simulink model "IdealScheme_soft_start"  (R2021b)
settings: Solver=VariableStepAuto  StartTime=0.0  StopTime=10  RelTol=1e-3
libraries: spsDiodeLib x7, spsMeanLib x5, spsSeriesRLCBranchLib x4, spsCurrentMeasurementLib x2, spsVoltageMeasurementLib x2, spsDCMachineLib x1, spsDCVoltageSourceLib x1, spsGroundLib x1, spsIGBTLib x1, slpidlib x1, spsThreePhaseSourceLib x1, spspowerguiLib x1
settings Model: Creator=kkaya674  LastModifiedBy=kkaya674
settings SolverCC: ZeroCrossAlgorithm=Adaptive
settings DebuggingCC: IgnoredZcDiagnostic=none

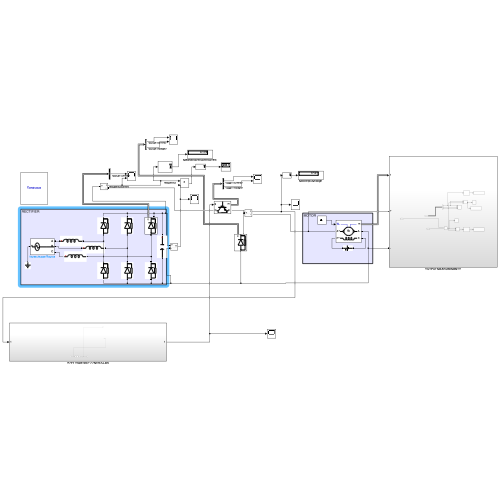
[thumbnail: Simulink's stored preview of the top-level diagram]
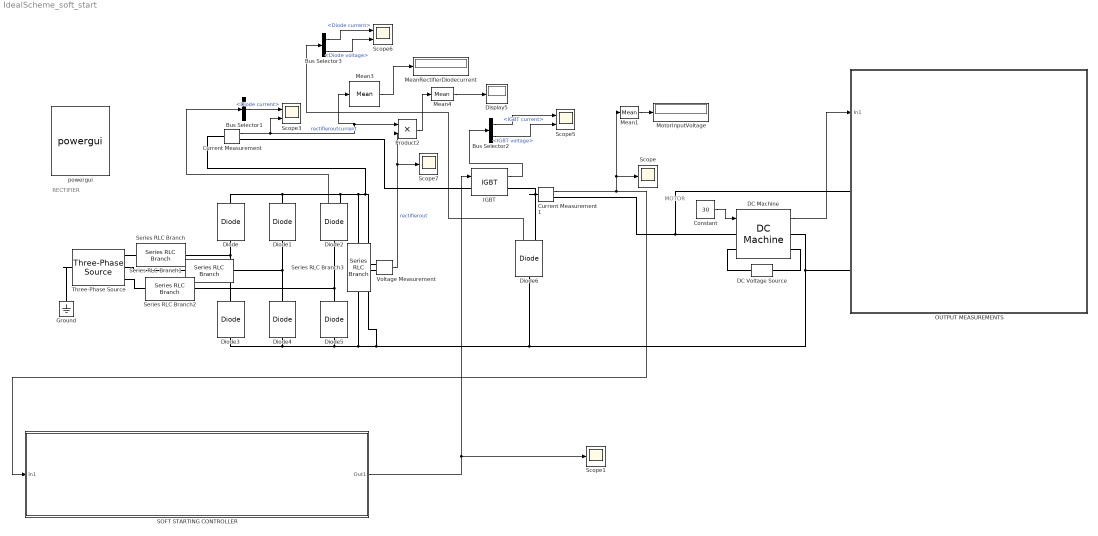
== system IdealScheme_soft_start ==
  note: MOTOR
  note: RECTIFIER
  Bus Selector1 : BusSelector  OutputSignals=Diode current
  Bus Selector2 : BusSelector  OutputSignals=IGBT current,IGBT voltage
  Bus Selector3 : BusSelector  OutputSignals=Diode current,Diode voltage
  Constant : Constant  Value=30
  Current Measurement : spsCurrentMeasurementLib/Current Measurement  PhasorSimulation=off  OutputType=Complex  PSBequivalent=0
  Current Measurement1 : spsCurrentMeasurementLib/Current Measurement  PhasorSimulation=off  OutputType=Complex  PSBequivalent=0
  DC Machine : spsDCMachineLib/DC Machine  PresetModel=No  MechanicalLoad=Torque TL  FieldType=Wound  ShowDetailedParameters=on  MeasurementBus=off  RLa=[0.8 12.5e-3]  RLf=[210 23]  Laf=1.8  MachineConstant=Torque constant (N.m/A)  Ke=1.8  Kt=1.8  J=1  Bm=0  Tf=0  w0=0  Ifinit=1.04761904756944  TsPowergui=0  TsBlock=-1
  DC Voltage Source : spsDCVoltageSourceLib/DC Voltage Source  Amplitude=220  Measurements=None
  Diode{,1,3..5} (5 alike) : spsDiodeLib/Diode  Ron=0.001  Lon=0  Vf=0.8  IC=0  UseSnubber=0  Rs=500  Cs=250e-9  Measurements=off
  Diode2 : spsDiodeLib/Diode  Ron=0.001  Lon=0  Vf=0.8  IC=0  UseSnubber=0  Rs=500  Cs=250e-9  Measurements=on
  Diode6 : spsDiodeLib/Diode  Ron=0.001  Lon=0  Vf=0.8  IC=0  UseSnubber=0  Rs=500  Cs=250e-9  Measurements=on
  Display5 : Display
  Ground : spsGroundLib/Ground  LConnTagsString=a
  IGBT : spsIGBTLib/IGBT  Ron=0.001  Lon=0  Vf=1  Tf=1e-6  Tt=2e-6  IC=0  Rs=1e5  Cs=inf  Measurements=on
  Mean1 : spsMeanLib/Mean  Freq=60  Vinit=0  Ts=0
  Mean3 : spsMeanLib/Mean  Freq=50  Vinit=0  Ts=0
  Mean4 : spsMeanLib/Mean  Freq=50  Vinit=0  Ts=0
  MeanRectifierDiodecurrent : Display
  MotorInputVoltage : Display
  OUTPUT MEASUREMENTS : Subsystem
  Product2 : Product
  SOFT STARTING CONTROLLER : Subsystem
  Scope : Scope
  Scope1 : Scope
  Scope3 : Scope  NumInputPorts=2
  Scope5 : Scope  NumInputPorts=2
  Scope6 : Scope  NumInputPorts=2
  Scope7 : Scope
  Series RLC Branch : spsSeriesRLCBranchLib/Series RLC Branch  LConnTagsString=__new0  RConnTagsString=__new0  BranchType=L  Resistance=1  Inductance=0.05e-3  SetiL0=off  InitialCurrent=0  Capacitance=1e-6  Setx0=off  InitialVoltage=0  Measurements=None
  Series RLC Branch1 : spsSeriesRLCBranchLib/Series RLC Branch  LConnTagsString=__new0  RConnTagsString=__new0  BranchType=L  Resistance=1  Inductance=0.05e-3  SetiL0=off  InitialCurrent=0  Capacitance=1e-6  Setx0=off  InitialVoltage=0  Measurements=None
  Series RLC Branch2 : spsSeriesRLCBranchLib/Series RLC Branch  LConnTagsString=__new0  RConnTagsString=__new0  BranchType=L  Resistance=1  Inductance=0.05e-3  SetiL0=off  InitialCurrent=0  Capacitance=1e-6  Setx0=off  InitialVoltage=0  Measurements=None
  Series RLC Branch3 : spsSeriesRLCBranchLib/Series RLC Branch  LConnTagsString=__new0  RConnTagsString=__new0  BranchType=C  Resistance=1  Inductance=1e-3  SetiL0=off  InitialCurrent=0  Capacitance=470e-6  Setx0=off  InitialVoltage=0  Measurements=None
  Three-Phase Source : spsThreePhaseSourceLib/Three-Phase Source  InternalConnection=Yn  VoltagePhases=off  Voltage=166  PhaseAngle=0  Voltage_phases=[25e3 25e3 25e3]/sqrt(3)  PhaseAngles_phases=[0 -120 +120]  Frequency=50  NonIdealSource=off  SpecifyImpedance=off  Resistance=0.8929  Inductance=16.58e-3  ShortCircuitLevel=100e6  BaseVoltage=25e3  XRratio=7  BusType=swing  Pref=10e3  Qref=0  Prefabc=[10e3, 10e3, 10e3]  Qrefabc=[0, 0, 0]  Qmin=-inf  Qmax=inf
  Voltage Measurement : spsVoltageMeasurementLib/Voltage Measurement  PhasorSimulation=off  OutputType=Complex  PSBequivalent=0
  powergui : spspowerguiLib/powergui  Priority=1  SimulationMode=Continuous  SampleTime=50e-6  frequency=60  Iterations=50  frequencyindice=0  Pbase=100e6  ErrMax=1e-4  UnitsV=kV  UnitsW=MW  buscounter=0  FunctionMessages=off  echomessages=off  EnableUseOfTLC=off  CurrentSourceSwitches=off  DisableSnubberDevices=off  DisableRonSwitches=off  DisableVfSwitches=off  DisplayEquations=off  AutomaticDiscreteSolvers=off  SolverType=Tustin/Backward Euler (TBE)  Interpol=off  ExternalGateDelay=off  methode=off  Ts=100  x0status=blocks  SPID=on  SwTol=0  HookPort=off  NonlinearTolerance=1e-4  nMaxIteration=100  ContinueOnMaxIteration=off  RestoreLinks=warning  ResistiveCurrentMeasurement=off  Frange=[0:2:500]  Ylog=off  Xlog=on  ShowGrid=off  save=off  variable=ZData  structure=0  ZoomFFT=off  StartTime=0.0  cycles=1  DisplayStyle=1  fundamental=60  FreqAxis=off  MaxFrequency=1000  frequencyindicesteady=1  RmsSteady=1  display=off
  wires:
  Voltage Measurement/1 -> Scope7/1, Product2/2  "rectifierout"
  Mean1/1 -> MotorInputVoltage/1
  IGBT/1 -> Bus Selector2/1
  Bus Selector2/1 -> Scope5/1  "<IGBT current>"
  Bus Selector2/2 -> Scope5/2  "<IGBT voltage>"
  Diode6/1 -> Bus Selector3/1
  Bus Selector3/1 -> Scope6/1  "<Diode current>"
  Bus Selector3/2 -> Scope6/2  "<Diode voltage>"
  Constant/1 -> DC Machine/1
  Diode2/1 -> Bus Selector1/1
  Bus Selector1/1 -> Scope3/1  "<Diode current>"
  Current Measurement/1 -> Scope3/2, Mean3/1, Product2/1  "rectifieroutcurrent"
  Mean3/1 -> MeanRectifierDiodecurrent/1
  Product2/1 -> Mean4/1
  Mean4/1 -> Display5/1
  Current Measurement1/1 -> Mean1/1, Scope/1, SOFT STARTING CONTROLLER/1(In1)
  DC Machine/1 -> OUTPUT MEASUREMENTS/1(In1)
  SOFT STARTING CONTROLLER/1(Out1) -> Scope1/1, IGBT/1
  connections:
  Diode3/RConn1 -- Series RLC Branch/RConn1 -- Diode/LConn1
  Diode4/RConn1 -- Series RLC Branch1/RConn1 -- Diode1/LConn1
  Diode5/RConn1 -- Series RLC Branch2/RConn1 -- Diode2/LConn1
  Current Measurement1/RConn1 -- OUTPUT MEASUREMENTS/LConn1 -- DC Machine/LConn1
  Diode/RConn1 -- Series RLC Branch3/LConn1 -- Voltage Measurement/LConn1 -- Current Measurement/LConn1 -- Diode2/RConn1 -- Diode1/RConn1
  Three-Phase Source/LConn1 -- Ground/LConn1
  DC Voltage Source/RConn1 -- DC Machine/LConn2
  DC Voltage Source/LConn1 -- DC Machine/RConn2
  IGBT/RConn1 -- Current Measurement1/LConn1 -- Diode6/RConn1
  IGBT/LConn1 -- Current Measurement/RConn1
  Three-Phase Source/RConn1 -- Series RLC Branch/LConn1
  Three-Phase Source/RConn2 -- Series RLC Branch1/LConn1
  Three-Phase Source/RConn3 -- Series RLC Branch2/LConn1
  Diode6/LConn1 -- OUTPUT MEASUREMENTS/LConn2 -- DC Machine/RConn1 -- Voltage Measurement/LConn2 -- Series RLC Branch3/RConn1 -- Diode4/LConn1 -- Diode3/LConn1 -- Diode5/LConn1

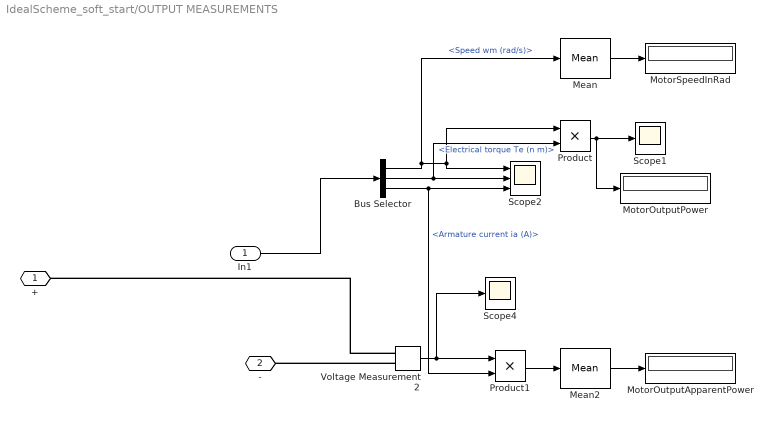
== system IdealScheme_soft_start/OUTPUT MEASUREMENTS ==
  In1 : Inport
  Bus Selector : BusSelector  OutputSignals=Speed wm (rad/s),Electrical torque Te (n m),Armature current ia (A)
  Mean : spsMeanLib/Mean  Freq=60  Vinit=0  Ts=0
  Mean2 : spsMeanLib/Mean  Freq=50  Vinit=0  Ts=0
  MotorOutputApparentPower : Display
  MotorOutputPower : Display
  MotorSpeedInRad : Display
  Product : Product
  Product1 : Product
  Scope1 : Scope
  Scope2 : Scope  NumInputPorts=3
  Scope4 : Scope
  Voltage Measurement2 : spsVoltageMeasurementLib/Voltage Measurement  PhasorSimulation=off  OutputType=Complex  PSBequivalent=0
  + : PMIOPort  Side=Left
  - : PMIOPort  Port=2  Side=Left
  wires:
  Voltage Measurement2/1 -> Product1/1, Scope4/1
  Bus Selector/2 -> Product/2, Scope2/2  "<Electrical torque Te (n m)>"
  In1/1 -> Bus Selector/1
  Mean/1 -> MotorSpeedInRad/1
  Product/1 -> MotorOutputPower/1, Scope1/1
  Product1/1 -> Mean2/1
  Bus Selector/1 -> Mean/1, Scope2/1, Product/1  "<Speed wm (rad/s)>"
  Mean2/1 -> MotorOutputApparentPower/1
  Bus Selector/3 -> Product1/2, Scope2/3  "<Armature current ia (A)>"
  connections:
  Voltage Measurement2/LConn2 -- -/RConn1
  Voltage Measurement2/LConn1 -- +/RConn1

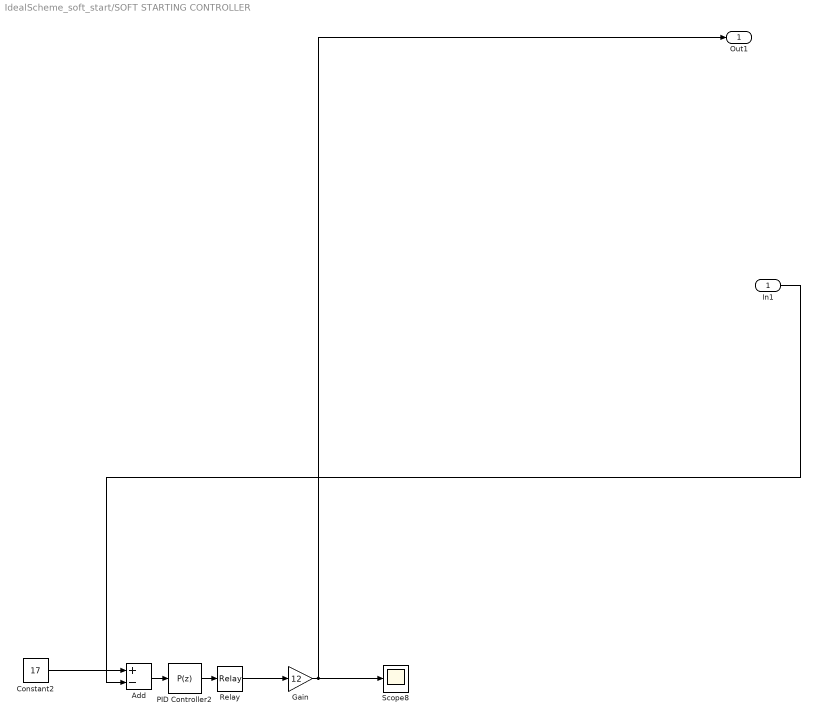
== system IdealScheme_soft_start/SOFT STARTING CONTROLLER ==
  In1 : Inport
  Add : Sum  Inputs=+-
  Constant2 : Constant  Value=17
  Gain : Gain  Gain=12
  PID Controller2 : slpidlib/PID Controller  Controller=P  Form=Parallel  TimeDomain=Discrete-time  UseExternalTs=off  SampleTime=-1  IntegratorMethod=Forward Euler  FilterMethod=Forward Euler  ControllerParametersSource=internal  P=1  I=0  D=0  UseFilter=on  N=100  TunerSelectOption=Transfer Function Based (PID Tuner App)  InitialConditionSource=internal  InitialConditionForIntegrator=0  InitialConditionForFilter=0  DifferentiatorICPrevScaledInput=0  ExternalReset=none  TrackingMode=off  Kt=1  LimitOutput=off  SatLimitsSource=internal  UpperSaturationLimit=inf  LowerSaturationLimit=-inf  LinearizeAsGain=on  AntiWindupMode=none  Kb=1  POutMin=[]  POutMax=[]  IOutMin=[]  IOutMax=[]  DOutMin=[]  DOutMax=[]  NOutMin=[]  NOutMax=[]  SumOutMin=[]  SumOutMax=[]  SaturationOutMin=[]  SaturationOutMax=[]  PParamMin=[]  PParamMax=[]  IParamMin=[]  IParamMax=[]  DParamMin=[]  DParamMax=[]  NParamMin=[]  NParamMax=[]  KbParamMin=[]  KbParamMax=[]  KtParamMin=[]  KtParamMax=[]  KbOutMin=[]  KbOutMax=[]  KtOutMin=[]  KtOutMax=[]  IntegratorOutMin=[]  IntegratorOutMax=[]  FilterOutMin=[]  FilterOutMax=[]  SumI1OutMin=[]  SumI1OutMax=[]  SumI2OutMin=[]  SumI2OutMax=[]  SumI3OutMin=[]  SumI3OutMax=[]  SumI4OutMin=[]  SumI4OutMax=[]  SumDOutMin=[]  SumDOutMax=[]  DifferentiatorOutMin=[]  DifferentiatorOutMax=[]  FilterDiffOutCoefMin=[]  FilterDiffOutCoefMax=[]  ReciprocalOutMin=[]  ReciprocalOutMax=[]  SumDenOutMin=[]  SumDenOutMax=[]  SumNumOutMin=[]  SumNumOutMax=[]  DivideOutMin=[]  DivideOutMax=[]  UdiffTsProdOutMin=[]  UdiffTsProdOutMax=[]  NTsProdOutMin=[]  NTsProdOutMax=[]  UintegralTsProdOutMin=[]  UintegralTsProdOutMax=[]  UngainTsProdOutMin=[]  UngainTsProdOutMax=[]  IntegratorContinuousStateAttributes=''  IntegratorStateMustResolveToSignalObject=off  IntegratorRTWStateStorageClass=Auto  FilterContinuousStateAttributes=''  FilterStateMustResolveToSignalObject=off  FilterRTWStateStorageClass=Auto  ParallelPVariant=InternalParameters  IdealPVariant=Disabled  IVariant=Disabled  DVariant=Disabled  IntegratorVariant=Disabled  SatVariant=Disabled  AWVariant=Disabled  PCopyVariant=Disabled  TRVariant=Disabled  FdbkBlocksVariant=Forward  IdealPFdbkVariant=Disabled  SatFdbkVariant=Disabled  DerivativeFilterVariant=Disabled  NVariant=Disabled  NCopyVariant=Disabled_SignalSpec  FilterICVariant=Disabled  IntegratorICVariant=Disabled  ExternalResetVariant=Disabled  TRSumVariant=Passthrough  SumFdbkVariant=Disabled  SumVariant=Passthrough_P  TsampFilterVariant=InternalTs  TsampNgainVariant=Passthrough  TsampIntegralVariant=Disabled_SignalSpec  ExternalSaturationOutDataTypeStr=Inherit: Same as second input
  Relay : Relay  OnSwitchValue=1  OffSwitchValue=-1
  Scope8 : Scope
  Out1 : Outport
  wires:
  Add/1 -> PID Controller2/1
  Relay/1 -> Gain/1
  Constant2/1 -> Add/1
  PID Controller2/1 -> Relay/1
  In1/1 -> Add/2
  Gain/1 -> Out1/1, Scope8/1
